simulink model "ASM_Team_Project_2025_SystemArchitecture"  (R2024b)
settings: Solver=VariableStepAuto  StartTime=0.0  StopTime=10.0  RelTol=1e-3
settings Model: Creator=samuel  LastModifiedBy=samuel

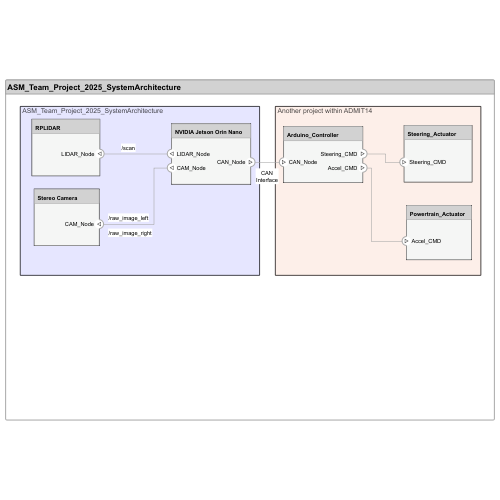
[thumbnail: Simulink's stored preview of the top-level diagram]
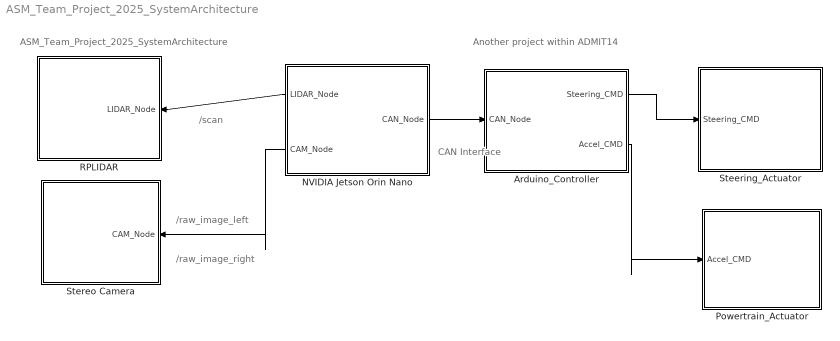
== system ASM_Team_Project_2025_SystemArchitecture ==
  note: CAN
      | Interface
  note: ASM_Team_Project_2025_SystemArchitecture
  note: Another project within ADMIT14
  note: /raw_image_right
  note: /raw_image_left
  note: /scan
  "Arduino_Controller " : Subsystem
      settings: PortSchema="{\"entries\":[{\"content\":{\"headerSize\":26,\"margin\":15,\"minimumSpacing\":25,\"sides\":[{\"content\":{\"connectorIds\":[\"In1\"]},\"type\":\"ConnectorPlacement.EquallySpacedRectSide\",\"uuid\":\"54c05843-4f2a-453c-a22a-ccdefaccabab\"},{\"content\":{\"connectorIds\":[\"Out1\",\"Out2\"],\"side\":\"RIGHT\"},\"type\":\"ConnectorPlacement.EquallySpacedRectSide\",\"uuid\":\"506f3d92-e40c-46ca-adf8-20501061295a\"},{\"content\":{\"side\":\"TOP\"},\"type\":\"ConnectorPlacement.EquallySpacedRectSide\",\"uuid\":\"72c9af18-5e8e-42b2-8264-de453ad24cde\"}]},\"type\":\"ConnectorPlacement.EquallySpacedConnector\",\"uuid\":\"ff460f51-5f3f-4ac3-9ade-ea7f16629e2f\"}],\"packageUris\":[\"http://schema.mathworks.com/mf0/Connector/R2020b\"],\"version\":\"1.0\"}"
  NVIDIA Jetson Orin Nano : Subsystem
      settings: PortSchema="{\"entries\":[{\"content\":{\"headerSize\":26,\"margin\":15,\"minimumSpacing\":25,\"sides\":[{\"content\":{\"connectorIds\":[\"Out2\",\"Out3\"]},\"type\":\"ConnectorPlacement.EquallySpacedRectSide\",\"uuid\":\"54c05843-4f2a-453c-a22a-ccdefaccabab\"},{\"content\":{\"connectorIds\":[\"Out1\"],\"side\":\"RIGHT\"},\"type\":\"ConnectorPlacement.EquallySpacedRectSide\",\"uuid\":\"506f3d92-e40c-46ca-adf8-20501061295a\"},{\"content\":{\"side\":\"TOP\"},\"type\":\"ConnectorPlacement.EquallySpacedRectSide\",\"uuid\":\"72c9af18-5e8e-42b2-8264-de453ad24cde\"}]},\"type\":\"ConnectorPlacement.EquallySpacedConnector\",\"uuid\":\"ff460f51-5f3f-4ac3-9ade-ea7f16629e2f\"}],\"packageUris\":[\"http://schema.mathworks.com/mf0/Connector/R2020b\"],\"version\":\"1.0\"}"
  Powertrain_Actuator : Subsystem
      settings: PortSchema="{\"entries\":[{\"content\":{\"headerSize\":26,\"margin\":15,\"minimumSpacing\":25,\"sides\":[{\"content\":{\"connectorIds\":[\"In1\"]},\"type\":\"ConnectorPlacement.EquallySpacedRectSide\",\"uuid\":\"54c05843-4f2a-453c-a22a-ccdefaccabab\"},{\"content\":{\"side\":\"RIGHT\"},\"type\":\"ConnectorPlacement.EquallySpacedRectSide\",\"uuid\":\"506f3d92-e40c-46ca-adf8-20501061295a\"},{\"content\":{\"side\":\"TOP\"},\"type\":\"ConnectorPlacement.EquallySpacedRectSide\",\"uuid\":\"72c9af18-5e8e-42b2-8264-de453ad24cde\"}]},\"type\":\"ConnectorPlacement.EquallySpacedConnector\",\"uuid\":\"ff460f51-5f3f-4ac3-9ade-ea7f16629e2f\"}],\"packageUris\":[\"http://schema.mathworks.com/mf0/Connector/R2020b\"],\"version\":\"1.0\"}"
  RPLIDAR : Subsystem
      settings: PortSchema="{\"entries\":[{\"content\":{\"headerSize\":26,\"margin\":15,\"minimumSpacing\":25,\"sides\":[{\"content\":{},\"type\":\"ConnectorPlacement.EquallySpacedRectSide\",\"uuid\":\"54c05843-4f2a-453c-a22a-ccdefaccabab\"},{\"content\":{\"connectorIds\":[\"In1\"],\"side\":\"RIGHT\"},\"type\":\"ConnectorPlacement.EquallySpacedRectSide\",\"uuid\":\"506f3d92-e40c-46ca-adf8-20501061295a\"},{\"content\":{\"side\":\"TOP\"},\"type\":\"ConnectorPlacement.EquallySpacedRectSide\",\"uuid\":\"72c9af18-5e8e-42b2-8264-de453ad24cde\"}]},\"type\":\"ConnectorPlacement.EquallySpacedConnector\",\"uuid\":\"ff460f51-5f3f-4ac3-9ade-ea7f16629e2f\"}],\"packageUris\":[\"http://schema.mathworks.com/mf0/Connector/R2020b\"],\"version\":\"1.0\"}"
  Steering_Actuator : Subsystem
      settings: PortSchema="{\"entries\":[{\"content\":{\"headerSize\":26,\"margin\":15,\"minimumSpacing\":25,\"sides\":[{\"content\":{\"connectorIds\":[\"In1\"]},\"type\":\"ConnectorPlacement.EquallySpacedRectSide\",\"uuid\":\"54c05843-4f2a-453c-a22a-ccdefaccabab\"},{\"content\":{\"side\":\"RIGHT\"},\"type\":\"ConnectorPlacement.EquallySpacedRectSide\",\"uuid\":\"506f3d92-e40c-46ca-adf8-20501061295a\"},{\"content\":{\"side\":\"TOP\"},\"type\":\"ConnectorPlacement.EquallySpacedRectSide\",\"uuid\":\"72c9af18-5e8e-42b2-8264-de453ad24cde\"}]},\"type\":\"ConnectorPlacement.EquallySpacedConnector\",\"uuid\":\"ff460f51-5f3f-4ac3-9ade-ea7f16629e2f\"}],\"packageUris\":[\"http://schema.mathworks.com/mf0/Connector/R2020b\"],\"version\":\"1.0\"}"
  "Stereo Camera " : Subsystem
      settings: PortSchema="{\"entries\":[{\"content\":{\"headerSize\":26,\"margin\":15,\"minimumSpacing\":25,\"sides\":[{\"content\":{},\"type\":\"ConnectorPlacement.EquallySpacedRectSide\",\"uuid\":\"54c05843-4f2a-453c-a22a-ccdefaccabab\"},{\"content\":{\"connectorIds\":[\"In1\"],\"side\":\"RIGHT\"},\"type\":\"ConnectorPlacement.EquallySpacedRectSide\",\"uuid\":\"506f3d92-e40c-46ca-adf8-20501061295a\"},{\"content\":{\"side\":\"TOP\"},\"type\":\"ConnectorPlacement.EquallySpacedRectSide\",\"uuid\":\"72c9af18-5e8e-42b2-8264-de453ad24cde\"}]},\"type\":\"ConnectorPlacement.EquallySpacedConnector\",\"uuid\":\"ff460f51-5f3f-4ac3-9ade-ea7f16629e2f\"}],\"packageUris\":[\"http://schema.mathworks.com/mf0/Connector/R2020b\"],\"version\":\"1.0\"}"
  wires:
  NVIDIA Jetson Orin Nano/2(LIDAR_Node) -> RPLIDAR/1(LIDAR_Node)
  NVIDIA Jetson Orin Nano/3(CAM_Node) -> "Stereo Camera "/1(CAM_Node)
  NVIDIA Jetson Orin Nano/1(CAN_Node) -> "Arduino_Controller "/1(CAN_Node)
  "Arduino_Controller "/1(Steering_CMD) -> Steering_Actuator/1(Steering_CMD)
  "Arduino_Controller "/2(Accel_CMD) -> Powertrain_Actuator/1(Accel_CMD)

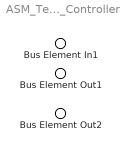
== system ASM_Team_Project_2025_SystemArchitecture/Arduino_Controller  ==
  Bus Element In1 : Inport  PortName=CAN_Node
  Bus Element Out1 : Outport  PortName=Steering_CMD
  Bus Element Out2 : Outport  Port=2  PortName=Accel_CMD

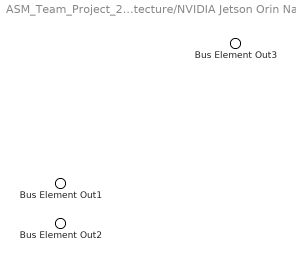
== system ASM_Team_Project_2025_SystemArchitecture/NVIDIA Jetson Orin Nano ==
  Bus Element Out3 : Outport  PortName=CAN_Node
  Bus Element Out1 : Outport  Port=2  PortName=LIDAR_Node
  Bus Element Out2 : Outport  Port=3  PortName=CAM_Node

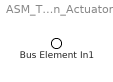
== system ASM_Team_Project_2025_SystemArchitecture/Powertrain_Actuator ==
  Bus Element In1 : Inport  PortName=Accel_CMD

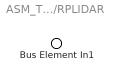
== system ASM_Team_Project_2025_SystemArchitecture/RPLIDAR ==
  Bus Element In1 : Inport  PortName=LIDAR_Node

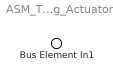
== system ASM_Team_Project_2025_SystemArchitecture/Steering_Actuator ==
  Bus Element In1 : Inport  PortName=Steering_CMD

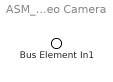
== system ASM_Team_Project_2025_SystemArchitecture/Stereo Camera  ==
  Bus Element In1 : Inport  PortName=CAM_Node
